simulink model "sxem"  (R2015b)
settings: Solver=VariableStepAuto  StartTime=0.0  StopTime=0.5  RelTol=1e-3
settings Model: Creator=hohotulca  LastModifiedBy=hohotulca

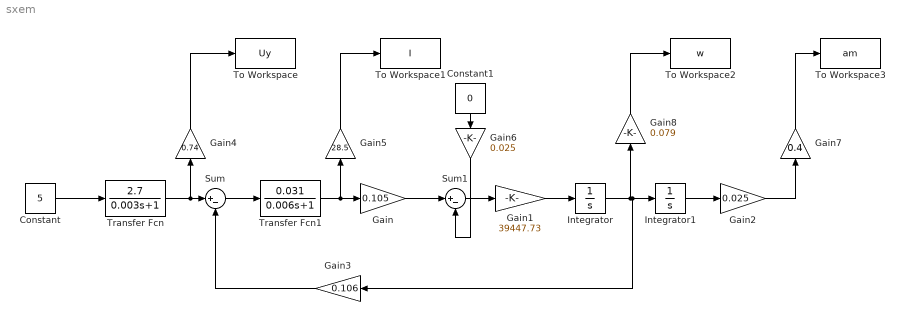
== system sxem ==
  Constant : Constant  Value=5
  Constant1 : Constant  Value=0
  Gain : Gain  Gain=0.105
  Gain1 : Gain  Gain=39447.73
  Gain2 : Gain  Gain=0.025
  Gain3 : Gain  Gain=0.106
  Gain4 : Gain  Gain=0.74
  Gain5 : Gain  Gain=28.5
  Gain6 : Gain  Gain=0.025
  Gain7 : Gain  Gain=0.4
  Gain8 : Gain  Gain=0.079
  Integrator : Integrator
  Integrator1 : Integrator
  Sum : Sum  Inputs=|+-
  Sum1 : Sum  Inputs=|+-
  To Workspace : ToWorkspace  VariableName=Uy  SaveFormat=Timeseries  SampleTime=-1
  To Workspace1 : ToWorkspace  VariableName=I  SaveFormat=Timeseries  SampleTime=-1
  To Workspace2 : ToWorkspace  VariableName=w  SaveFormat=Timeseries  SampleTime=-1
  To Workspace3 : ToWorkspace  VariableName=am  SaveFormat=Timeseries  SampleTime=-1
  Transfer Fcn : TransferFcn  Numerator=[2.7]  Denominator=[0.003 1]
  Transfer Fcn1 : TransferFcn  Numerator=[0.031]  Denominator=[0.006 1]
  wires:
  Constant/1 -> Transfer Fcn/1
  Transfer Fcn/1 -> Gain4/1, Sum/1
  Sum/1 -> Transfer Fcn1/1
  Transfer Fcn1/1 -> Gain5/1, Gain/1
  Gain/1 -> Sum1/1
  Sum1/1 -> Gain1/1
  Gain1/1 -> Integrator/1
  Integrator/1 -> Gain3/1, Integrator1/1, Gain8/1
  Integrator1/1 -> Gain2/1
  Gain3/1 -> Sum/2
  Gain4/1 -> To Workspace/1
  Gain5/1 -> To Workspace1/1
  Gain6/1 -> Sum1/2
  Constant1/1 -> Gain6/1
  Gain8/1 -> To Workspace2/1
  Gain7/1 -> To Workspace3/1
  Gain2/1 -> Gain7/1
